simulink subsystem "MPC14_nlpsol"  (R2022b)
settings: Solver=VariableStepAuto  StartTime=0.0  StopTime=10.0  RelTol=1e-3
undefined symbols (not defined in the file): param_global, param_jointspace_ct, param_MPC14, param_robot, param_weight_init
settings Model: Creator=emu  LastModifiedBy=emu
settings OptimizationCC: ReuseModelBlockBuffer=on

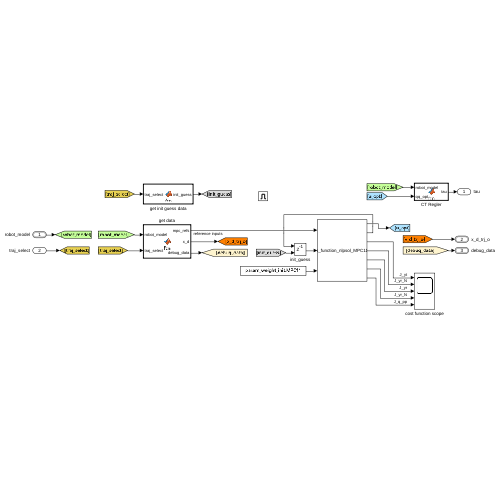
[thumbnail: Simulink's stored preview of the top-level diagram]
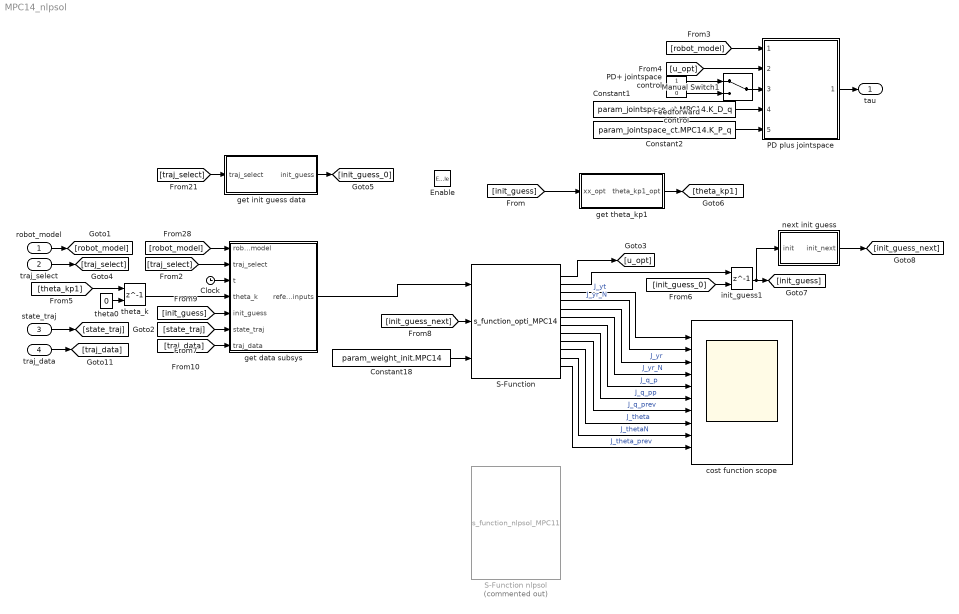
== system MPC14_nlpsol ==
  robot_model : Inport  OutDataTypeStr=Bus: robot_model
  traj_select : Inport  Port=2
  state_traj : Inport  Port=3  OutDataTypeStr=Bus: state_traj_bus
  traj_data : Inport  Port=4  OutDataTypeStr=Bus: traj_data_bus
  Enable : EnablePort
  Clock : Clock
  Constant1 : Constant  Value=param_jointspace_ct.MPC14.K_D_q
  Constant18 : Constant  Value=param_weight_init.MPC14  VectorParams1D=off
  Constant2 : Constant  Value=param_jointspace_ct.MPC14.K_P_q
  Feedforward control : Constant  Value=0
  Manual Switch1 : ManualSwitch
  PD plus jointspace : Subsystem  ReferencedSubsystem=closed_loop_kin_mpc_pdplus_control_refsys
  PD+ jointspace control : Constant
  S-Function : S-Function  FunctionName=s_function_opti_MPC14  SFunctionModules='MPC14'  SFunctionDeploymentMode=off  EnableBusSupport=off
  S-Function nlpsol : S-Function  Commented=on  FunctionName=s_function_nlpsol_MPC11  Parameters='s_functions/fr3_no_hand_6dof/MPC11.casadi', 'MPC11'  SFunctionModules='MPC11'  SFunctionDeploymentMode=off  EnableBusSupport=off
  cost function scope : Scope  NumInputPorts=10
  get data subsys : Subsystem
  get init guess data : MATLAB Function  TreatAsAtomicUnit=on
  get theta_kp1 : MATLAB Function  TreatAsAtomicUnit=on
  init_guess1 : Delay  DelayLength=1  InitialConditionSource=Input port  InitialCondition=1  SampleTime=param_global.Ta
      settings: InputPortMap=u0,p4
  next init guess : MATLAB Function  TreatAsAtomicUnit=on
  theta0 : Constant  Value=0  VectorParams1D=off
  theta_k : Delay  DelayLength=1  InitialConditionSource=Input port  InitialCondition=1
      settings: InputPortMap=u0,p4
  tau : Outport
  wires:
  [traj_data] -> get data subsys/7(traj_data)
  traj_data/1 -> [traj_data]
  [init_guess_next] -> S-Function/2
  next init guess/1(init_next) -> [init_guess_next]
  [init_guess] -> get data subsys/5(init_guess)
  S-Function/10 -> cost function scope/8  "J_theta"
  [init_guess] -> get theta_kp1/1(xx_opt)
  S-Function/2 -> init_guess1/1
  init_guess1/1 -> next init guess/1(init), [init_guess]
  [init_guess_0] -> init_guess1/2
  theta_k/1 -> get data subsys/4(theta_k)
  [theta_kp1] -> theta_k/1
  theta0/1 -> theta_k/2
  get theta_kp1/1(theta_kp1_opt) -> [theta_kp1]
  get data subsys/1(reference inputs) -> S-Function/1
  Clock/1 -> get data subsys/3(t)
  [traj_select] -> get data subsys/2(traj_select)
  [robot_model] -> get data subsys/1(robot_model)
  S-Function/9 -> cost function scope/7  "J_q_prev"
  S-Function/8 -> cost function scope/6  "J_q_pp"
  S-Function/1 -> [u_opt]
  S-Function/5 -> cost function scope/3  "J_yr"
  S-Function/3 -> cost function scope/1  "J_yt"
  Constant18/1 -> S-Function/3
  get init guess data/1(init_guess) -> [init_guess_0]
  robot_model/1 -> [robot_model]
  S-Function/4 -> cost function scope/2  "J_yr_N"
  traj_select/1 -> [traj_select]
  S-Function/6 -> cost function scope/4  "J_yr_N"
  PD plus jointspace/1 -> tau/1
  [traj_select] -> get init guess data/1(traj_select)
  S-Function/7 -> cost function scope/5  "J_q_p"
  state_traj/1 -> [state_traj]
  [state_traj] -> get data subsys/6(state_traj)
  Manual Switch1/1 -> PD plus jointspace/3
  Constant1/1 -> PD plus jointspace/4
  Constant2/1 -> PD plus jointspace/5
  [u_opt] -> PD plus jointspace/2
  PD+ jointspace control/1 -> Manual Switch1/1
  Feedforward control/1 -> Manual Switch1/2
  [robot_model] -> PD plus jointspace/1
  S-Function/11 -> cost function scope/9  "J_thetaN"
  S-Function/12 -> cost function scope/10  "J_theta_prev"

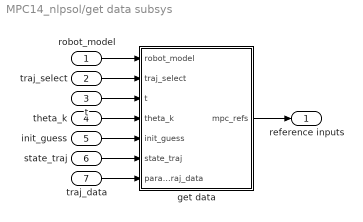
== system MPC14_nlpsol/get data subsys ==
  robot_model : Inport  OutDataTypeStr=Bus: robot_model
  traj_select : Inport  Port=2
  t : Inport  Port=3
  theta_k : Inport  Port=4
  init_guess : Inport  Port=5
  state_traj : Inport  Port=6  OutDataTypeStr=Bus: state_traj_bus
  traj_data : Inport  Port=7  OutDataTypeStr=Bus: traj_data_bus
  get data : MATLAB Function  TreatAsAtomicUnit=on
  reference inputs : Outport
  wires:
  state_traj/1 -> get data/6(state_traj)
  robot_model/1 -> get data/1(robot_model)
  get data/1(mpc_refs) -> reference inputs/1
  traj_select/1 -> get data/2(traj_select)
  t/1 -> get data/3(t)
  theta_k/1 -> get data/4(theta_k)
  init_guess/1 -> get data/5(init_guess)
  traj_data/1 -> get data/7(param_traj_data)

== matlab function MPC14_nlpsol/get data subsys/get data ==
  settings: updateMethod=DISCRETE  sampleTime=param_global.Ta
  data: mpc_refs output; robot_model input Bus: robot_model; traj_select input; t input; theta_k input; init_guess input; param_robot parameter; state_traj input Bus: state_traj_bus; param_MPC14 parameter; param_traj_data input
function mpc_refs = fcn(robot_model, traj_select, t, theta_k, init_guess, param_robot, state_traj, param_MPC14, param_traj_data)
persistent cnt;
persistent run_flag;

if(isempty(cnt))
    cnt = 1;
    run_flag = 0;
end

n_red = param_robot.n_red;
n_indices = param_robot.n_indices;
N_MPC = param_MPC14.N;

% Parameters
q    = robot_model.q;      % generalized coordinates
q_p  = robot_model.q_p;  % time derivative of generalized coordinates

x_k = [q(n_indices); q_p(n_indices)];

%% Reference out
N_theta = N_MPC;
N_u = n_red*N_MPC;
N_q = n_red * (N_MPC+1);
N_x = 2*N_q;
q_k_prev = init_guess(1+N_u : N_u+N_q);
theta_k_prev = init_guess(1+N_u+N_x: N_u+N_x+N_theta);
mpc_refs = [x_k(:); t; q_k_prev(:); theta_k_prev(:)];

[run_flag, cnt] = update_traj_cnt(state_traj, run_flag, cnt, param_traj_data.N);

== matlab function MPC14_nlpsol/get init guess data ==
  data: traj_select input; param_MPC14_init_guess parameter; init_guess output
function init_guess   = fcn(traj_select, param_MPC14_init_guess)

init_guess = param_MPC14_init_guess.init_guess(traj_select,:);

== matlab function MPC14_nlpsol/get theta_kp1 ==
  data: xx_opt input; theta_kp1_opt output; param_robot parameter; param_MPC14 parameter
function theta_kp1_opt = fcn(xx_opt, param_robot, param_MPC14)

N_MPC = param_MPC14.N;
n_red = param_robot.n_red;

N_u = n_red*N_MPC;
N_x = 2*n_red*(N_MPC+1);
theta_kp1_idx = 2 + N_u + N_x;
if size(xx_opt, 2) ~= 0 && size(xx_opt, 1) ~= 1
    theta_kp1_opt = xx_opt(theta_kp1_idx);
else
    theta_kp1_opt = 0;
end

== matlab function MPC14_nlpsol/next init guess ==
  data: init input; init_next output; param_MPC14 parameter; param_robot parameter; param_global parameter
function init_next = fcn(init, param_MPC14, param_robot, param_global)
param_MPC = param_MPC14;

Ta = param_global.Ta;
dt_arr = param_MPC.int_times;
N_MPC = param_MPC.N;
n_red = param_robot.n_red;
N_u = n_red * N_MPC;
N_x = (2*n_red)*(N_MPC+1);
N_theta = N_MPC;

N = 0;

init_next = init';

%% u next
u_idx = N + [1:N_u];       N = N + length(u_idx);
u_idx_2d = reshape(u_idx, n_red, (N_MPC));
u_idx_2d(:, 1:end-1) = u_idx_2d(:, 2:end);
u_init = init(u_idx_2d);

du = (u_init(:, 2:end) - u_init(:, 1:end-1))./dt_arr(1:end-1);
u_next = u_init(:, 1:end-1) + du * Ta;

u_idx_m1 = u_idx_2d(:, 1:end-1);
init_next(u_idx_m1) = u_next;
%% x next
x_idx = N + [1:N_x];       N = N + length(x_idx);
x_idx_2d = reshape(x_idx, 2*n_red, (N_MPC+1));
x_idx_2d(:, 1:end-1) = x_idx_2d(:, 2:end);
x_init = init(x_idx_2d);

dx = (x_init(:, 2:end) - x_init(:, 1:end-1))./dt_arr;
x_next = x_init(:, 1:end-1) + dx * Ta;

x_idx_m1 = x_idx_2d(:, 1:end-1);
init_next(x_idx_m1) = x_next;

%% theta next
%theta_idx = N + [1:N_theta];       N = N + length(theta_idx);
%theta_next = init(theta_idx) + Ta;
%init_next(theta_idx) = theta_next;
